simulink model "Green_Led_Harness"  (R2022b)
settings: Solver=VariableStepAuto  StartTime=0.0  StopTime=50.0  RelTol=1e-3
settings Model: Creator=chiar  LastModifiedBy=chiar
settings ConfigComp: CovEnable=on  RecordCoverage=on  CovModelRefEnable=on

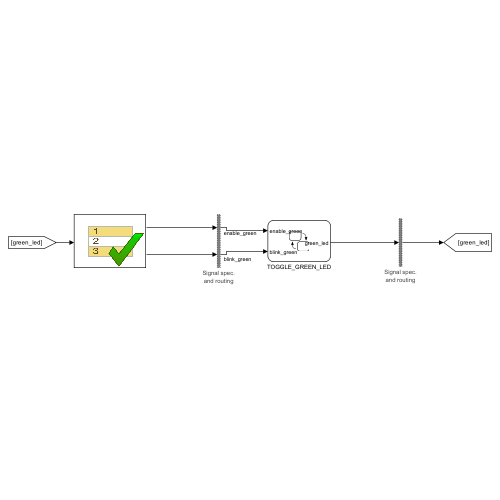
[thumbnail: Simulink's stored preview of the top-level diagram]
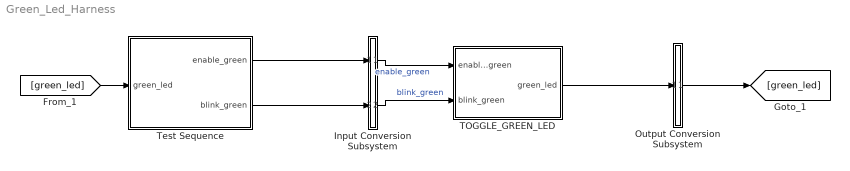
== system Green_Led_Harness ==
  Input Conversion Subsystem : Subsystem  Tag=__SLT_ICS__  Description=|
      | Signal spec.
      | and routing
      settings: AttributesFormatString=%<Description>
  Output Conversion Subsystem : Subsystem  Tag=__SLT_OCS__  Description=|
      | Signal spec.
      | and routing
      settings: AttributesFormatString=%<Description>
  TOGGLE_GREEN_LED : Stateflow chart  TreatAsAtomicUnit=on
  Test Sequence : Test Sequence  TreatAsAtomicUnit=on
  wires:
  Test Sequence/1(enable_green) -> Input Conversion Subsystem/1(Inport_1)
  Test Sequence/2(blink_green) -> Input Conversion Subsystem/2(Inport_2)
  [green_led] -> Test Sequence/1(green_led)
  Output Conversion Subsystem/1(Outport_1) -> [green_led]
  Input Conversion Subsystem/1(Outport_1) -> TOGGLE_GREEN_LED/1(enable_green)  "enable_green"
  Input Conversion Subsystem/2(Outport_2) -> TOGGLE_GREEN_LED/2(blink_green)  "blink_green"
  TOGGLE_GREEN_LED/1(green_led) -> Output Conversion Subsystem/1(Inport_1)

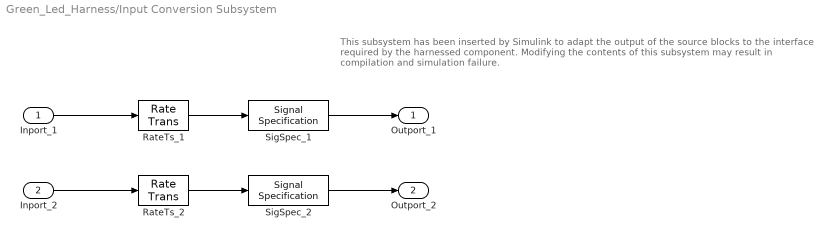
== system Green_Led_Harness/Input Conversion Subsystem ==
  note: This subsystem has been inserted by Simulink to adapt the output of the source blocks to the interface required by the harnessed component.
      |  Modifying the contents of this subsystem may result in compilation and simulation failure.
  Inport_1 : Inport
  Inport_2 : Inport  Port=2
  RateTs_1 : RateTransition  OutPortSampleTime=[0, 1]
  RateTs_2 : RateTransition  OutPortSampleTime=[0, 1]
  SigSpec_1 : SignalSpecification  OutDataTypeStr=boolean  Dimensions=[1]  SampleTime=[0, 1]
  SigSpec_2 : SignalSpecification  OutDataTypeStr=boolean  Dimensions=[1]  SampleTime=[0, 1]
  Outport_1 : Outport
  Outport_2 : Outport  Port=2
  wires:
  SigSpec_1/1 -> Outport_1/1
  RateTs_1/1 -> SigSpec_1/1
  Inport_1/1 -> RateTs_1/1
  SigSpec_2/1 -> Outport_2/1
  RateTs_2/1 -> SigSpec_2/1
  Inport_2/1 -> RateTs_2/1

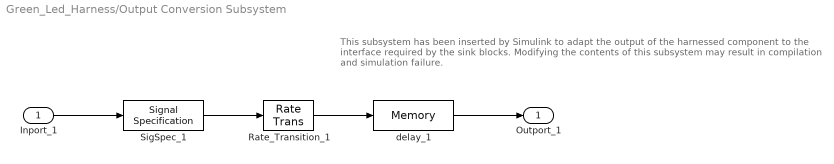
== system Green_Led_Harness/Output Conversion Subsystem ==
  note: This subsystem has been inserted by Simulink to adapt the output of the harnessed component to the interface required by the sink blocks.
      |  Modifying the contents of this subsystem may result in compilation and simulation failure.
  Inport_1 : Inport
  Rate_Transition_1 : RateTransition  OutPortSampleTimeOpt=Inherit
  SigSpec_1 : SignalSpecification  OutDataTypeStr=boolean  Dimensions=[1]
  delay_1 : Memory
  Outport_1 : Outport
  wires:
  Inport_1/1 -> SigSpec_1/1
  SigSpec_1/1 -> Rate_Transition_1/1
  Rate_Transition_1/1 -> delay_1/1
  delay_1/1 -> Outport_1/1

== stateflow chart Green_Led_Harness/TOGGLE_GREEN_LED ==
  state TOGGLE_GREEN
    state SWITCH
      state SWITCH_OFF
        en: green_led = OFF
      state SWITCH_ON
        en: green_led = ON
      (default) -> SWITCH_OFF
      SWITCH_OFF -> SWITCH_ON : [enable_green == ON]
      SWITCH_ON -> SWITCH_OFF : [enable_green == OFF]
    state BLINKING
      state BLINKING_ON
        en: green_led = ON
      state BLINKING_OFF
        en: green_led = OFF
      (default) -> BLINKING_ON
      BLINKING_OFF -> BLINKING_ON : [after(TGREEN, sec)]
      BLINKING_ON -> BLINKING_OFF : [after(TGREEN, sec)]
    (default) -> SWITCH
    SWITCH -> BLINKING : [blink_green == ON]
    BLINKING -> SWITCH : [blink_green == OFF]
  data: TGREEN constant double =1; OFF constant boolean =0; ON constant boolean =1; enable_green input boolean; green_led output boolean; blink_green input boolean

== stateflow chart Green_Led_Harness/Test Sequence ==
  settings: updateMethod=DISCRETE  sampleTime=0.2
  state Scenario_1
    state INIT
      %% Initialize data outputs.
      enable_green = false;
      blink_green = false;
      n = 0;
      verify(green_led == false);
    state LED_ON
      enable_green = true;
      blink_green = false;
    state CHECK_LED_ON
      verify(green_led == true);
    state LED_OFF
      enable_green = false;
      blink_green = false;
    state CHECK_LED_OFF
      verify(green_led == false);
    state ACTIVATE_BLINKING
      enable_green = false;
      blink_green = true;
    state BLINKING
      settings: description=|
          | NON MODIFICARE
          | IL VALORE DI n!!!!!
          | Aumentandolo si
          | introducono leggeri
          | ritardi che a lungo
          | andare portano a
          | risultati errati. Questo
          | è dovuto alla frequenza
          | di lampeggio molto
          | bassa.
      state BLINKING_ON
        verify(green_led == true);
      state BLINKING_INTERMEDIATE
        n = n+1;
        settings: description=|
            | n = n+1 viene usato
            | per fare in modo che
            | si esca dallo step
            | mentre siamo in
            | BLINKING_ON. È
            | stato messo qui perché
            | altrove avrebbe
            | introdotto un ritardo
            | causando un errore
            | nella verify.
      state BLINKING_OFF
        verify(green_led == false);
      (default) -> Scenario_1.BLINKING.BLINKING_ON
      (junction 262) -> Scenario_1.BLINKING.BLINKING_ON
      (junction 264) -> (junction 262)
      Scenario_1.BLINKING.BLINKING_OFF -> (junction 264) : [
          | after(0.8, sec)
          | ]
      Scenario_1.BLINKING.BLINKING_ON -> Scenario_1.BLINKING.BLINKING_INTERMEDIATE : [
          | after(0.8, sec)
          | ]
      Scenario_1.BLINKING.BLINKING_INTERMEDIATE -> Scenario_1.BLINKING.BLINKING_OFF : [
          | after(0.4, sec)
          | ]
    state TURNING_OFF
      enable_green = false;
      blink_green = false;
    state FINAL
      verify(green_led == false);
    (default) -> Scenario_1.INIT
    Scenario_1.INIT -> Scenario_1.LED_ON : [
        | after(2, sec)
        | ]
    Scenario_1.LED_ON -> Scenario_1.CHECK_LED_ON : [
        | after(2, sec)
        | ]
    Scenario_1.CHECK_LED_ON -> LED_OFF : [
        | after(2, sec)
        | ]
    LED_OFF -> CHECK_LED_OFF : [
        | after(2, sec)
        | ]
    CHECK_LED_OFF -> Scenario_1.ACTIVATE_BLINKING : [
        | after(2, sec)
        | ]
    Scenario_1.ACTIVATE_BLINKING -> Scenario_1.BLINKING : [
        | after(0.4,sec)
        | ]
    Scenario_1.BLINKING -> Scenario_1.TURNING_OFF : [
        | n == 6
        | ]
    Scenario_1.TURNING_OFF -> Scenario_1.FINAL : [
        | after(2, sec)
        | ]
  state Scenario_2
    state INIT
      %% Initialize data outputs.
      enable_green = false;
      blink_green = false;
      verify(green_led == false);
    state LED_ON
      enable_green = true;
      blink_green = false;
      n = 0;
    state CHECK_LED_ON
      verify(green_led == true);
    state ACTIVATE_BLINKING
      blink_green = true;
    state BLINKING
      state BLINKING_ON
        verify(green_led == true);
      state BLINKING_OFF
        verify(green_led == false);
      state BLINKING_INTERMEDIATE
        n = n+1;
        settings: description=|
            | n = n+1 viene usato
            | per fare in modo che
            | si esca dallo step
            | mentre siamo in
            | BLINKING_OFF. È
            | stato messo lì perché
            | altrove avrebbe
            | introdotto un ritardo
            | causando un errore
            | nella verify.
      Scenario_2.BLINKING.BLINKING_INTERMEDIATE -> (junction 282) : [
          | after(0.8, sec)
          | ]
      (default) -> Scenario_2.BLINKING.BLINKING_ON
      (junction 280) -> Scenario_2.BLINKING.BLINKING_ON
      Scenario_2.BLINKING.BLINKING_ON -> Scenario_2.BLINKING.BLINKING_OFF : [
          | after(0.8, sec)
          | ]
      Scenario_2.BLINKING.BLINKING_OFF -> Scenario_2.BLINKING.BLINKING_INTERMEDIATE : [
          | after(0.4, sec)
          | ]
      (junction 282) -> (junction 280)
    state TURNING_OFF
      enable_green = true;
      blink_green = false;
    state FINAL
      verify(green_led == true);
    (default) -> Scenario_2.INIT
    Scenario_2.INIT -> Scenario_2.LED_ON : [
        | after(2, sec)
        | ]
    Scenario_2.LED_ON -> Scenario_2.CHECK_LED_ON : [
        | after(2, sec)
        | ]
    Scenario_2.ACTIVATE_BLINKING -> Scenario_2.BLINKING : [
        | after(0.5,sec)
        | ]
    Scenario_2.BLINKING -> Scenario_2.TURNING_OFF : [
        | n == 6
        | ]
    Scenario_2.TURNING_OFF -> Scenario_2.FINAL : [
        | after(2, sec)
        | ]
    Scenario_2.CHECK_LED_ON -> Scenario_2.ACTIVATE_BLINKING : [
        | after(2, sec)
        | ]
  (default) -> Scenario_1 [order 1] : [Active_Scenario_Index == 1]
  (default) -> Scenario_2 [order 2] : {assert(Active_Scenario_Index == 2,'The value of Scenario Parameter ''Active_Scenario_Index'' is not valid. Use the index of the scenario to specify it.')}
  data: green_led input boolean size=[1]; enable_green output boolean size=[1]; blink_green output boolean size=[1]; n local; Active_Scenario_Index parameter =2
